simulink library "Valeo_Simulink_Library_EC"  (R2017b)
settings: Solver=ode45  StartTime=0.0  StopTime=10.0  RelTol=1e-3  EnableMultiTasking=on
undefined symbols (not defined in the file): A, B, C, Count_Max, D, InitValue, j, ke, kf, kt, L, Length, MaxIniVal, MaxVal, MinVal, NumBits1, NumBits2, P, p0, Q, R, Simulink_Library, Ts, x0
libraries: Valeo_Simulink_Library_EC x9, simulink x8, fixpt_dtprop x4
(part 2 of 3)

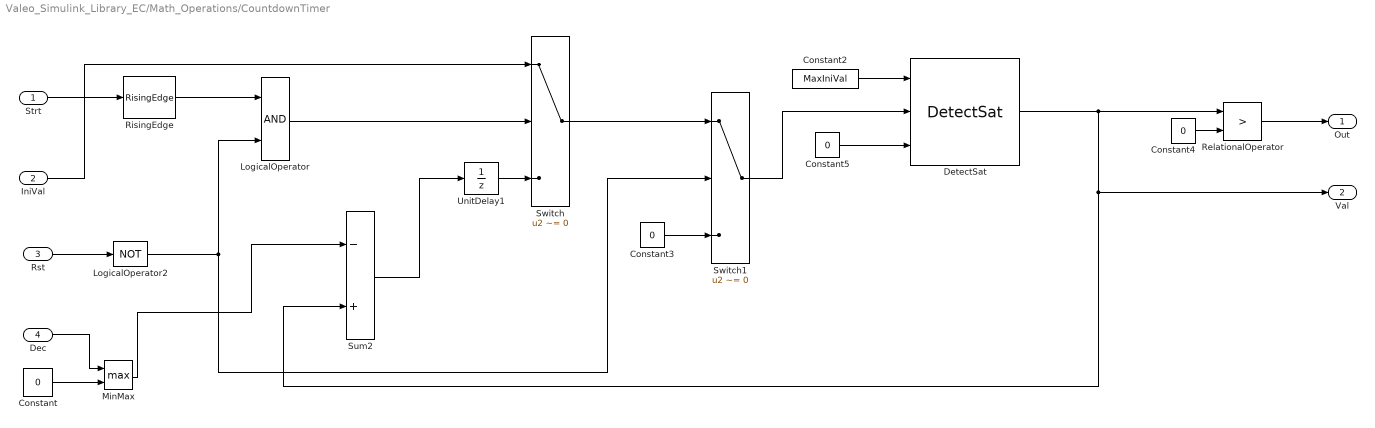
== system Valeo_Simulink_Library_EC/Math_Operations/CountdownTimer ==
  Strt : Inport
  IniVal : Inport  Port=2
  Rst : Inport  Port=3
  Dec : Inport  Port=4
  Constant : Constant  Value=0  OutDataTypeStr=Inherit: Inherit via back propagation
  Constant2 : Constant  Value=MaxIniVal  OutDataTypeStr=Inherit: Inherit via back propagation  SampleTime=-1
  Constant3 : Constant  Value=0  OutDataTypeStr=Inherit: Inherit via back propagation  SampleTime=-1
  Constant4 : Constant  Value=0  OutDataTypeStr=Inherit: Inherit via back propagation  SampleTime=-1
  Constant5 : Constant  Value=0  OutDataTypeStr=Inherit: Inherit via back propagation  SampleTime=-1
  DetectSat : Valeo_Simulink_Library_EC/Signal_Operations/DetectSat  FlagHitMax=off  FlagHitMin=off  FlagOut=on  FlagRevThr=off  EnableRevThreshold=No  LibType=Simulink_Library
  LogicalOperator : Logic  OutDataTypeStr=boolean
  LogicalOperator2 : Logic  Operator=NOT  Inputs=3  OutDataTypeStr=boolean
  MinMax : MinMax  Function=max  Inputs=2  InputSameDT=on
  RelationalOperator : RelationalOperator  Operator=>  OutDataTypeStr=boolean  RndMeth=Nearest  InputSameDT=on
  RisingEdge : Valeo_Simulink_Library_EC/Signal_Operations/RisingEdge  INIT=0
  Sum2 : Sum  Inputs=-+  OutDataTypeStr=Inherit: Inherit via back propagation  RndMeth=Nearest  SaturateOnIntegerOverflow=on  InputSameDT=on
  Switch : Switch  Tag=struct('comment',struct('text','','placement',1),'logdata',struct('maxnumvals',inf,'plotchannels',[],'loggingmode',3,'channels',1),'output',struct('variable','','description','','name','$S_$B','width',1,'address','','max',NaN,'min',NaN,'class','default','type','CONTINUOUS','scaling','','lsb',1,'offset',0,'arb',0,'freeze',1,'unit','','autoscalingmode',1,'lowerheadroom',1,'upperheadroom',1,'headroomunit','bit','keepdatatype',1,'checkmin',0,'checkmax',0,'castoutput',0,'show',0),'threshold',struct('variable','','description','','name','$S_$B_threshold','width',1,'address','','max',NaN,'min',NaN,'class','default','type','CONTINUOUS','scaling','','lsb',1,'offset',0,'arb',0,'freeze',1,'unit','','keepdatatype',1,'value','0','scalar',0,'criteria',3),'scalingvalid',0,'date',733087.49614628474,'inheritscaling',0)  Criteria=u2 ~= 0  OutDataTypeStr=Inherit: Inherit via back propagation  RndMeth=Nearest  SaturateOnIntegerOverflow=on  InputSameDT=on
      settings: AttributesFormatString=threshold=%<threshold>\nCriteria : %<Criteria>
  Switch1 : Switch  Tag=struct('comment',struct('text','','placement',1),'logdata',struct('maxnumvals',inf,'plotchannels',[],'loggingmode',3,'channels',1),'output',struct('variable','','description','','name','$S_$B','width',1,'address','','max',NaN,'min',NaN,'class','default','type','CONTINUOUS','scaling','','lsb',1,'offset',0,'arb',0,'freeze',1,'unit','','autoscalingmode',1,'lowerheadroom',1,'upperheadroom',1,'headroomunit','bit','keepdatatype',1,'checkmin',0,'checkmax',0,'castoutput',0,'show',0),'threshold',struct('variable','','description','','name','$S_$B_threshold','width',1,'address','','max',NaN,'min',NaN,'class','default','type','CONTINUOUS','scaling','','lsb',1,'offset',0,'arb',0,'freeze',1,'unit','','keepdatatype',1,'value','0','scalar',0,'criteria',3),'scalingvalid',0,'date',733087.49614628474,'inheritscaling',0)  Criteria=u2 ~= 0  RndMeth=Nearest  SaturateOnIntegerOverflow=on  InputSameDT=on
      settings: AttributesFormatString=threshold=%<threshold>\nCriteria : %<Criteria>
  UnitDelay1 : UnitDelay  SampleTime=-1
      settings: AttributesFormatString=%<Name>\nTe = %<SampleTime>\nIni=%<X0>
  Out : Outport
  Val : Outport  Port=2
  wires:
  Constant/1 -> MinMax/2
  Constant5/1 -> DetectSat/3
  Constant4/1 -> RelationalOperator/2
  UnitDelay1/1 -> Switch/3
  DetectSat/1 -> Val/1, Sum2/2, RelationalOperator/1
  IniVal/1 -> Switch/1
  LogicalOperator/1 -> Switch/2
  Rst/1 -> LogicalOperator2/1
  RelationalOperator/1 -> Out/1
  Strt/1 -> RisingEdge/1
  RisingEdge/1 -> LogicalOperator/1
  LogicalOperator2/1 -> Switch1/2, LogicalOperator/2
  Constant3/1 -> Switch1/3
  Switch/1 -> Switch1/1
  Dec/1 -> MinMax/1
  Constant2/1 -> DetectSat/1
  Switch1/1 -> DetectSat/2
  MinMax/1 -> Sum2/1
  Sum2/1 -> UnitDelay1/1

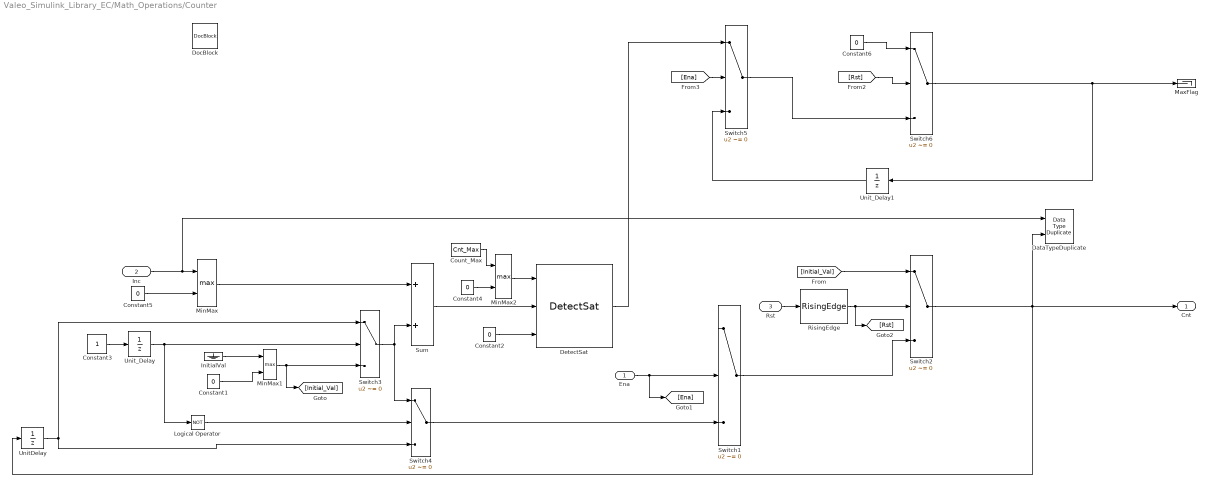
== system Valeo_Simulink_Library_EC/Math_Operations/Counter ==
  Ena : Inport  OutDataTypeStr=boolean
  Inc : Inport  Port=2
  Rst : Inport  Port=3
  Constant{1..2,4..6} (5 alike) : Constant  Value=0  OutDataTypeStr=Inherit: Inherit via back propagation  SampleTime=-1
  Constant3 : Constant  OutDataTypeStr=boolean  SampleTime=-1
  Count_Max : Constant  Value=Cnt_Max
  DataTypeDuplicate : DataTypeDuplicate
  DetectSat : Valeo_Simulink_Library_EC/Signal_Operations/DetectSat  RequirementInfo={} %GIDa_9bb61fc0_0d7a_4d30_bf11_8496912d343b  FlagHitMax=on  FlagHitMin=off  FlagOut=on  FlagRevThr=off  EnableRevThreshold=Yes  LibType=Simulink_Library
  DocBlock : simulink/Model-Wide Utilities/DocBlock  DocumentType=Text
      content=|
      | Block Name: Counter
      |
      | Description:
      | Count up block optional inputs and outputs as per the needed application.
      | "Ena" inport and "Cnt" outport are mandatory.
      | "Inc", "Rst", "InitialVal" and "Count_Max" are optional inports.
      | "MaxFlag" is an optional outport.
      | If "Inc" is not selected from the mask, default increment step is 1.
      | If "Rst" is not selected from the mask, the port is grounded.
      | If "InitialVal" is not selected from the mask, default initial value is 0.
      | If "Count_Max" is not selected from the mask, the value has to be entered
      | from the mask itself as a parameter.
      | If "MaxFlag" is not selected from the mask, the port is terminated.
      |
      | Requirements Document:VIAS_T02_15_019_Valeo_Simulink_Library_SRS
      |                       Section:5.1.4
      |
      | Last Edit made by: sahmed1 on 17/3/2019
      |
      | Block Version: 1.1
  InitialVal : Ground
  Logical Operator : Logic  Operator=NOT  AllPortsSameDT=off  OutDataTypeStr=boolean
  MaxFlag : Terminator
  MinMax : MinMax  RequirementInfo={} %GIDa_05f1e69c_f4c8_4dbb_8851_ae441f19c864  Function=max  Inputs=2  OutDataTypeStr=Inherit: Inherit via back propagation  ZeroCross=off  SaturateOnIntegerOverflow=on  InputSameDT=on
  MinMax1 : MinMax  Function=max  Inputs=2  OutDataTypeStr=Inherit: Inherit via back propagation  ZeroCross=off  SaturateOnIntegerOverflow=on  InputSameDT=on
  MinMax2 : MinMax  Function=max  Inputs=2  OutDataTypeStr=Inherit: Inherit via back propagation  ZeroCross=off  SaturateOnIntegerOverflow=on  InputSameDT=on
  RisingEdge : Valeo_Simulink_Library_EC/Signal_Operations/RisingEdge  RequirementInfo={} %GIDa_9731123e_4d8d_47b4_b498_60fb13b5864c  INIT=0
  Sum : Sum  RequirementInfo={} %GIDa_8f895930_75b4_4d04_b64c_37162e5979c7  OutDataTypeStr=Inherit: Inherit via back propagation  SaturateOnIntegerOverflow=on  InputSameDT=on
  Switch1 : Switch  Tag=struct('comment',struct('text','','placement',1),'logdata',struct('maxnumvals',inf,'plotchannels',[],'loggingmode',3,'channels',1),'output',struct('variable','','description','','name','$S_$B','width',1,'address','','max',NaN,'min',NaN,'class','default','type','CONTINUOUS','scaling','','lsb',1,'offset',0,'arb',0,'freeze',1,'unit','','autoscalingmode',1,'lowerheadroom',1,'upperheadroom',1,'headroomunit','bit','keepdatatype',1,'checkmin',0,'checkmax',0,'castoutput',0,'show',0),'threshold',struct('variable','','description','','name','$S_$B_threshold','width',1,'address','','max',NaN,'min',NaN,'class','default','type','CONTINUOUS','scaling','','lsb',1,'offset',0,'arb',0,'freeze',1,'unit','','keepdatatype',1,'value','0','scalar',0,'criteria',3),'scalingvalid',0,'date',733087.49614628474,'inheritscaling',0)  RequirementInfo={} %GIDa_3188b40d_7524_43cd_a4e7_8fa433184620  Criteria=u2 ~= 0  ZeroCross=off  InputSameDT=on
      settings: AttributesFormatString=threshold=%<threshold>\nCriteria : %<Criteria>
  Switch2 : Switch  Tag=struct('comment',struct('text','','placement',1),'logdata',struct('maxnumvals',inf,'plotchannels',[],'loggingmode',3,'channels',1),'output',struct('variable','','description','','name','$S_$B','width',1,'address','','max',NaN,'min',NaN,'class','default','type','CONTINUOUS','scaling','','lsb',1,'offset',0,'arb',0,'freeze',1,'unit','','autoscalingmode',1,'lowerheadroom',1,'upperheadroom',1,'headroomunit','bit','keepdatatype',1,'checkmin',0,'checkmax',0,'castoutput',0,'show',0),'threshold',struct('variable','','description','','name','$S_$B_threshold','width',1,'address','','max',NaN,'min',NaN,'class','default','type','CONTINUOUS','scaling','','lsb',1,'offset',0,'arb',0,'freeze',1,'unit','','keepdatatype',1,'value','0','scalar',0,'criteria',3),'scalingvalid',0,'date',733087.49614628474,'inheritscaling',0)  RequirementInfo={} %GIDa_e3ab621a_27e3_4b82_bf67_d379718e39ab  Criteria=u2 ~= 0  OutDataTypeStr=Inherit: Inherit via back propagation  ZeroCross=off  InputSameDT=on
      settings: AttributesFormatString=threshold=%<threshold>\nCriteria : %<Criteria>
  Switch3 : Switch  RequirementInfo={} %GIDa_6adc28a8_417c_42d0_96f8_0bd9c0ac3dfc  Criteria=u2 ~= 0  RndMeth=Nearest  InputSameDT=on
      settings: AttributesFormatString=Cond=%<Criteria>\nThreshold=%<Threshold>
  Switch4 : Switch  RequirementInfo={} %GIDa_4bec96d5_6195_44e1_b82b_bfaee5774d71  Criteria=u2 ~= 0  RndMeth=Nearest  InputSameDT=on
      settings: AttributesFormatString=Cond=%<Criteria>\nThreshold=%<Threshold>
  Switch5 : Switch  Tag=struct('comment',struct('text','','placement',1),'logdata',struct('maxnumvals',inf,'plotchannels',[],'loggingmode',3,'channels',1),'output',struct('variable','','description','','name','$S_$B','width',1,'address','','max',NaN,'min',NaN,'class','default','type','CONTINUOUS','scaling','','lsb',1,'offset',0,'arb',0,'freeze',1,'unit','','autoscalingmode',1,'lowerheadroom',1,'upperheadroom',1,'headroomunit','bit','keepdatatype',1,'checkmin',0,'checkmax',0,'castoutput',0,'show',0),'threshold',struct('variable','','description','','name','$S_$B_threshold','width',1,'address','','max',NaN,'min',NaN,'class','default','type','CONTINUOUS','scaling','','lsb',1,'offset',0,'arb',0,'freeze',1,'unit','','keepdatatype',1,'value','0','scalar',0,'criteria',3),'scalingvalid',0,'date',733087.49614628474,'inheritscaling',0)  RequirementInfo={} %GIDa_5a250cc1_c600_4491_b832_9bb443b73e74  Criteria=u2 ~= 0  ZeroCross=off  InputSameDT=on
      settings: AttributesFormatString=threshold=%<threshold>\nCriteria : %<Criteria>
  Switch6 : Switch  Tag=struct('comment',struct('text','','placement',1),'logdata',struct('maxnumvals',inf,'plotchannels',[],'loggingmode',3,'channels',1),'output',struct('variable','','description','','name','$S_$B','width',1,'address','','max',NaN,'min',NaN,'class','default','type','CONTINUOUS','scaling','','lsb',1,'offset',0,'arb',0,'freeze',1,'unit','','autoscalingmode',1,'lowerheadroom',1,'upperheadroom',1,'headroomunit','bit','keepdatatype',1,'checkmin',0,'checkmax',0,'castoutput',0,'show',0),'threshold',struct('variable','','description','','name','$S_$B_threshold','width',1,'address','','max',NaN,'min',NaN,'class','default','type','CONTINUOUS','scaling','','lsb',1,'offset',0,'arb',0,'freeze',1,'unit','','keepdatatype',1,'value','0','scalar',0,'criteria',3),'scalingvalid',0,'date',733087.49614628474,'inheritscaling',0)  RequirementInfo={} %GIDa_72ede8d6_7b52_4ad1_ab42_e02456330975  Criteria=u2 ~= 0  OutDataTypeStr=Inherit: Inherit via back propagation  ZeroCross=off  InputSameDT=on
      settings: AttributesFormatString=threshold=%<threshold>\nCriteria : %<Criteria>
  UnitDelay : UnitDelay  SampleTime=-1
      settings: AttributesFormatString=%<Name>\nTe = %<SampleTime>\nIni=%<X0>
  Unit_Delay : UnitDelay  SampleTime=-1
  Unit_Delay1 : UnitDelay  SampleTime=-1
  Cnt : Outport  RequirementInfo={} %GIDa_ced6db0b_0aef_4b74_b197_441398289d0b
  wires:
  Switch5/1 -> Switch6/3
  Constant6/1 -> Switch6/1
  Unit_Delay1/1 -> Switch5/3
  [Ena] -> Switch5/2
  DetectSat/1 -> Switch5/1
  [Rst] -> Switch6/2
  Rst/1 -> RisingEdge/1
  ? -> Switch1/1
  Switch6/1 -> Unit_Delay1/1, MaxFlag/1
  Sum/1 -> DetectSat/2
  Count_Max/1 -> MinMax2/1
  MinMax2/1 -> DetectSat/1
  InitialVal/1 -> MinMax1/1
  MinMax1/1 -> Switch3/3, [Initial_Val]
  Constant1/1 -> MinMax1/2
  Constant4/1 -> MinMax2/2
  Switch1/1 -> Switch2/3
  MinMax/1 -> Sum/1
  Unit_Delay/1 -> Logical Operator/1, Switch3/2
  Constant3/1 -> Unit_Delay/1
  Switch3/1 -> Switch4/1, Sum/2
  Inc/1 -> MinMax/1, DataTypeDuplicate/1
  RisingEdge/1 -> Switch2/2, [Rst]
  Constant5/1 -> MinMax/2
  Constant2/1 -> DetectSat/3
  Ena/1 -> Switch1/2, [Ena]
  Switch4/1 -> Switch1/3
  Logical Operator/1 -> Switch4/2
  Switch2/1 -> DataTypeDuplicate/2, Cnt/1, UnitDelay/1
  UnitDelay/1 -> Switch4/3, Switch3/1
  [Initial_Val] -> Switch2/1

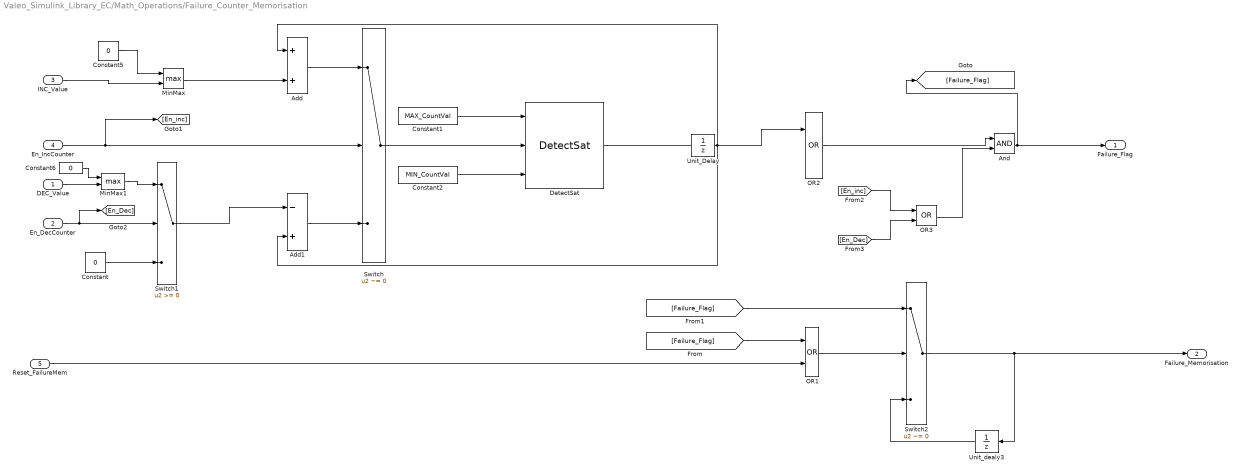
== system Valeo_Simulink_Library_EC/Math_Operations/Failure_Counter_Memorisation ==
  DEC_Value : Inport
  En_DecCounter : Inport  Port=2  OutDataTypeStr=boolean
  INC_Value : Inport  Port=3
  En_IncCounter : Inport  Port=4  OutDataTypeStr=boolean
  Reset_FailureMem : Inport  Port=5  OutDataTypeStr=boolean
  Add : Sum
  Add1 : Sum  Inputs=-+
  And : Logic  AllPortsSameDT=off  OutDataTypeStr=boolean
  Constant : Constant  Value=0  OutDataTypeStr=Inherit: Inherit via back propagation
  Constant1 : Constant  Value=MAX_CountVal
  Constant2 : Constant  Value=MIN_CountVal
  Constant5 : Constant  Value=0  OutDataTypeStr=Inherit: Inherit via back propagation
  Constant6 : Constant  Value=0  OutDataTypeStr=Inherit: Inherit via back propagation
  DetectSat : Valeo_Simulink_Library_EC/Signal_Operations/DetectSat  Description=DetectSat  RequirementInfo={} %GIDa_f7c90ce4_a1b3_4851_83d7_a18600e936e6  FlagHitMax=on  FlagHitMin=on  FlagOut=on  FlagRevThr=off  EnableRevThreshold=No  LibType=Simulink_Library
  MinMax : MinMax  Function=max  Inputs=2
  MinMax1 : MinMax  Function=max  Inputs=2
  OR1 : Logic  RequirementInfo={} %GIDa_04208e23_291f_48af_9c39_d5bad472f985  Operator=OR  AllPortsSameDT=off  OutDataTypeStr=boolean
  OR2 : Logic  RequirementInfo={} %GIDa_9651d414_1c4d_4a50_8930_c47158f8b0f5  Operator=OR  AllPortsSameDT=off  OutDataTypeStr=boolean
  OR3 : Logic  Operator=OR  AllPortsSameDT=off  OutDataTypeStr=boolean
  Switch : Switch  RequirementInfo={} %GIDa_288fa2ec_3de0_4803_93ac_92640899949d  Criteria=u2 ~= 0
  Switch1 : Switch
  Switch2 : Switch  RequirementInfo={} %GIDa_0183bc51_af57_411f_b819_c082a7e6d6c2  Criteria=u2 ~= 0
  Unit_Delay : UnitDelay  SampleTime=-1
  Unit_dealy3 : UnitDelay  SampleTime=-1
  Failure_Flag : Outport  Tag=AM,Out,1,0,Name,NC;CMP,Port,OutputWhenDisabled,InitialOutput;  OutDataTypeStr=boolean
      settings: AttributesFormatString=%<OutputWhenDisabled>\n%<InitialOutput>\n
  Failure_Memorisation : Outport  Port=2  OutDataTypeStr=boolean
  wires:
  [Failure_Flag] -> OR1/1
  [Failure_Flag] -> Switch2/1
  Unit_dealy3/1 -> Switch2/3
  OR1/1 -> Switch2/2
  Switch2/1 -> Unit_dealy3/1, Failure_Memorisation/1
  Reset_FailureMem/1 -> OR1/2
  En_IncCounter/1 -> Switch/2, [En_inc]
  MinMax/1 -> Add/2
  INC_Value/1 -> MinMax/2
  Add/1 -> Switch/1
  Unit_Delay/1 -> Add/1, Add1/2
  Switch1/1 -> Add1/1
  Constant/1 -> Switch1/3
  En_DecCounter/1 -> [En_Dec], Switch1/2
  MinMax1/1 -> Switch1/1
  Constant6/1 -> MinMax1/1
  DEC_Value/1 -> MinMax1/2
  Add1/1 -> Switch/3
  And/1 -> [Failure_Flag], Failure_Flag/1
  OR2/1 -> And/1
  OR3/1 -> And/2
  [En_Dec] -> OR3/2
  [En_inc] -> OR3/1
  Constant5/1 -> MinMax/1
  Constant2/1 -> DetectSat/3
  Constant1/1 -> DetectSat/1
  Switch/1 -> DetectSat/2
  DetectSat/1 -> OR2/1
  ? -> OR2/2
  ? -> Unit_Delay/1

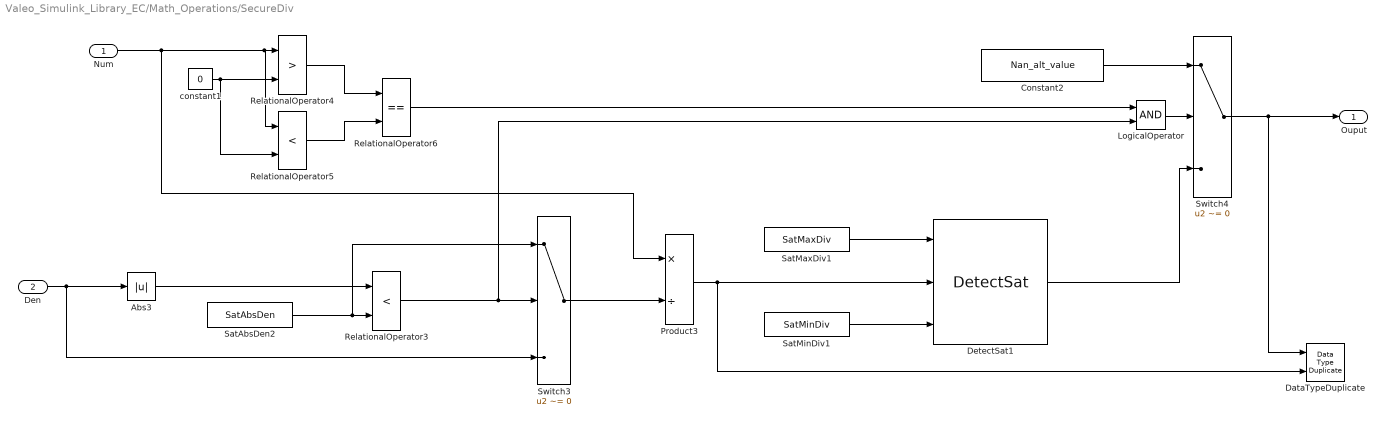
== system Valeo_Simulink_Library_EC/Math_Operations/SecureDiv ==
  Num : Inport
  Den : Inport  Port=2
  Abs3 : Abs  SaturateOnIntegerOverflow=on
  Constant2 : Constant  Value=Nan_alt_value  OutDataTypeStr=Inherit: Inherit via back propagation  SampleTime=-1  LockScale=on
  DataTypeDuplicate : DataTypeDuplicate
  DetectSat1 : Valeo_Simulink_Library_EC/Signal_Operations/DetectSat  FlagHitMax=off  FlagHitMin=off  FlagOut=on  FlagRevThr=off  EnableRevThreshold=No  LibType=Simulink_Library
  LogicalOperator : Logic  AllPortsSameDT=off  OutDataTypeStr=boolean
  Product3 : Product  Tag=struct('comment',struct('text','','placement',1),'logdata',struct('maxnumvals',inf,'plotchannels',[],'loggingmode',3,'channels',1),'output',struct('variable','','description','','name','$S_$B','width',1,'address','','max',NaN,'min',NaN,'class','default','type','CONTINUOUS','scaling','','lsb',1,'offset',0,'arb',0,'freeze',1,'unit','','autoscalingmode',1,'lowerheadroom',1,'upperheadroom',1,'headroomunit','bit','keepdatatype',1,'checkmin',0,'checkmax',0,'castoutput',0,'show',0),'inputs','**','exceptionhandling',1,'scalingvalid',0,'date',730486)  Inputs=*/  OutDataTypeStr=Inherit: Inherit via back propagation  RndMeth=Nearest  SaturateOnIntegerOverflow=on
  RelationalOperator3 : RelationalOperator  Operator=<  OutDataTypeStr=boolean  RndMeth=Nearest  InputSameDT=on
  RelationalOperator4 : RelationalOperator  Operator=>  OutDataTypeStr=boolean  RndMeth=Nearest  InputSameDT=on
  RelationalOperator5 : RelationalOperator  Operator=<  OutDataTypeStr=boolean  RndMeth=Nearest  InputSameDT=on
  RelationalOperator6 : RelationalOperator  Operator===  OutDataTypeStr=boolean  RndMeth=Nearest  InputSameDT=on
  SatAbsDen2 : Constant  Tag=struct('comment',struct('text','','placement',1),'output',struct('variable','','description','','name','$S_$B','width',1,'address','','max',NaN,'min',NaN,'class','default','type','CONTINUOUS','scaling','','lsb',1,'offset',0,'arb',0,'freeze',1,'unit','','keepdatatype',1,'value','1','tolerance',1,'castoutput',0,'show',0),'dt','inf','scalingvalid',0,'date',730486)  Value=SatAbsDen  OutDataTypeStr=Inherit: Inherit via back propagation  SampleTime=-1
  SatMaxDiv1 : Constant  Tag=struct('comment',struct('text','','placement',1),'output',struct('variable','','description','','name','$S_$B','width',1,'address','','max',NaN,'min',NaN,'class','default','type','CONTINUOUS','scaling','','lsb',1,'offset',0,'arb',0,'freeze',1,'unit','','keepdatatype',1,'value','1','tolerance',1,'castoutput',0,'show',0),'dt','inf','scalingvalid',0,'date',730486)  Value=SatMaxDiv  OutDataTypeStr=Inherit: Inherit via back propagation  SampleTime=-1
  SatMinDiv1 : Constant  Tag=struct('comment',struct('text','','placement',1),'output',struct('variable','','description','','name','$S_$B','width',1,'address','','max',NaN,'min',NaN,'class','default','type','CONTINUOUS','scaling','','lsb',1,'offset',0,'arb',0,'freeze',1,'unit','','keepdatatype',1,'value','1','tolerance',1,'castoutput',0,'show',0),'dt','inf','scalingvalid',0,'date',730486)  Value=SatMinDiv  OutDataTypeStr=Inherit: Inherit via back propagation  SampleTime=-1
  Switch3 : Switch  Tag=struct('comment',struct('text','','placement',1),'logdata',struct('maxnumvals',inf,'plotchannels',[],'loggingmode',3,'channels',1),'output',struct('variable','','description','','name','$S_$B','width',1,'address','','max',NaN,'min',NaN,'class','default','type','CONTINUOUS','scaling','','lsb',1,'offset',0,'arb',0,'freeze',1,'unit','','autoscalingmode',1,'lowerheadroom',1,'upperheadroom',1,'headroomunit','bit','keepdatatype',1,'checkmin',0,'checkmax',0,'castoutput',0,'show',0),'threshold',struct('variable','','description','','name','$S_$B_threshold','width',1,'address','','max',NaN,'min',NaN,'class','default','type','CONTINUOUS','scaling','','lsb',1,'offset',0,'arb',0,'freeze',1,'unit','','keepdatatype',1,'value','0','scalar',0,'criteria',3),'scalingvalid',0,'date',733087.49614628474,'inheritscaling',0)  Criteria=u2 ~= 0  SaturateOnIntegerOverflow=on  InputSameDT=on
      settings: AttributesFormatString=threshold=%<threshold>\nCriteria : %<Criteria>
  Switch4 : Switch  Criteria=u2 ~= 0  OutDataTypeStr=Inherit: Inherit via back propagation  RndMeth=Nearest  InputSameDT=on
  constant1 : Constant  Tag=struct('comment',struct('text','','placement',1),'output',struct('variable','','description','','name','$S_$B','width',1,'address','','max',NaN,'min',NaN,'class','default','type','CONTINUOUS','scaling','','lsb',1,'offset',0,'arb',0,'freeze',1,'unit','','keepdatatype',1,'value','1','tolerance',1,'castoutput',0,'show',0),'dt','inf','scalingvalid',0,'date',730486)  Value=0  OutDataTypeStr=Inherit: Inherit via back propagation  SampleTime=-1
  Ouput : Outport
  wires:
  DetectSat1/1 -> Switch4/3
  LogicalOperator/1 -> Switch4/2
  RelationalOperator6/1 -> LogicalOperator/1
  Switch4/1 -> Ouput/1, DataTypeDuplicate/1
  Constant2/1 -> Switch4/1
  RelationalOperator5/1 -> RelationalOperator6/2
  RelationalOperator4/1 -> RelationalOperator6/1
  constant1/1 -> RelationalOperator5/2, RelationalOperator4/2
  Num/1 -> RelationalOperator5/1, RelationalOperator4/1, Product3/1
  SatMaxDiv1/1 -> DetectSat1/1
  SatMinDiv1/1 -> DetectSat1/3
  Product3/1 -> DetectSat1/2, DataTypeDuplicate/2
  SatAbsDen2/1 -> RelationalOperator3/2, Switch3/1
  Switch3/1 -> Product3/2
  RelationalOperator3/1 -> Switch3/2, LogicalOperator/2
  Abs3/1 -> RelationalOperator3/1
  Den/1 -> Switch3/3, Abs3/1

== system Valeo_Simulink_Library_EC/Plant Models/Actuators ==
  BLDC : Subsystem  mask(VSL_BLDC){R=R, L=L, j=j, P=P, ke=ke, kt=kt, kf=kf, x0=x0}
      mask help: BLDC motor model simulates the machine speed, torque and stator currents stimulated by the phase to phase voltage and load torque, assuming trapezoidal back emf.
      mask Display:
      | plot(0,0,100,100)
      | patch(100*[0.88 0.93 0.94 0.99 0.98 0.94 0.9 0.88], 100*[0.11 0.01 0.01 0.11 0.11 0.026 0.11 0.11], [0 1 0])

== system Valeo_Simulink_Library_EC/Plant Models/Sensors ==

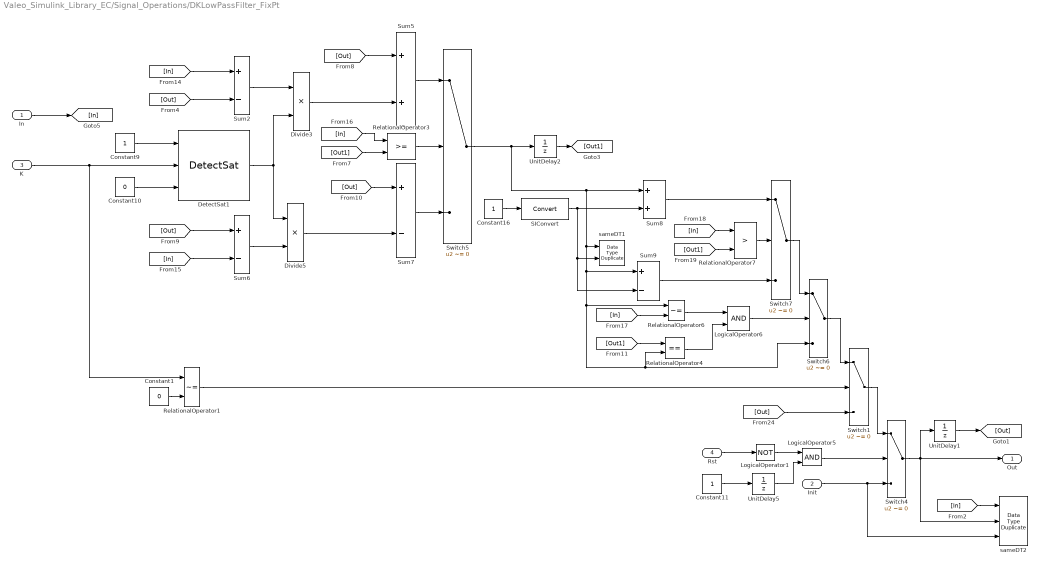
== system Valeo_Simulink_Library_EC/Signal_Operations/DKLowPassFilter_FixPt ==
  In : Inport  RequirementInfo={} %GIDa_0413d053_4ec8_42c5_b371_a8047b2200f3
  Init : Inport  RequirementInfo={} %GIDa_5872fcc3_05fb_45f2_9bed_09235c6b0cac  Port=2
  K : Inport  RequirementInfo={} %GIDa_98114ef1_cbe3_4be6_8894_0cd40cae6f0b  Port=3
  Rst : Inport  RequirementInfo={} %GIDa_1420b06f_654a_4f9a_a3af_ddfdee9c425a  Port=4
  Constant1 : Constant  Value=0  OutDataTypeStr=Inherit: Inherit via back propagation  SampleTime=-1
  Constant10 : Constant  RequirementInfo={} %GIDa_3973ca9d_f818_47df_80ed_9838d1273ef8  Value=0  OutDataTypeStr=Inherit: Inherit via back propagation  SampleTime=-1
  Constant11 : Constant  RequirementInfo={} %GIDa_d28a1eeb_ec69_477b_bb73_5596cd9e0263  OutDataTypeStr=boolean  SampleTime=-1
  Constant16 : Constant  RequirementInfo={} %GIDa_6d10a8d6_24a5_4fbd_9218_f05ddc57d3c3  OutDataTypeStr=uint8  SampleTime=-1
  Constant9 : Constant  RequirementInfo={} %GIDa_f21fb39a_79b6_494f_8e0c_3ee289bd9826  OutDataTypeStr=Inherit: Inherit via back propagation  SampleTime=-1
  DetectSat1 : Valeo_Simulink_Library_EC/Signal_Operations/DetectSat  RequirementInfo={} %GIDa_5313b4e0_40e1_4e21_9a31_65be49b89e34  FlagHitMax=off  FlagHitMin=off  FlagOut=on  FlagRevThr=off  EnableRevThreshold=No  LibType=Simulink_Library
  Divide3 : Product  Tag=struct('comment',struct('text','','placement',1),'logdata',struct('maxnumvals',inf,'plotchannels',[],'loggingmode',3,'channels',1),'output',struct('variable','','description','','name','$S_$B','width',1,'address','','max',NaN,'min',NaN,'class','default','type','CONTINUOUS','scaling','','lsb',1,'offset',0,'arb',0,'freeze',1,'unit','','autoscalingmode',1,'lowerheadroom',1,'upperheadroom',1,'headroomunit','bit','keepdatatype',1,'checkmin',0,'checkmax',0,'castoutput',0,'show',0),'inputs','**','exceptionhandling',1,'scalingvalid',0,'date',730486)  RequirementInfo={} %GIDa_0415ca49_d04f_4698_b9e2_db1e83986d60  Inputs=**  RndMeth=Simplest  SaturateOnIntegerOverflow=on
  Divide5 : Product  Tag=struct('comment',struct('text','','placement',1),'logdata',struct('maxnumvals',inf,'plotchannels',[],'loggingmode',3,'channels',1),'output',struct('variable','','description','','name','$S_$B','width',1,'address','','max',NaN,'min',NaN,'class','default','type','CONTINUOUS','scaling','','lsb',1,'offset',0,'arb',0,'freeze',1,'unit','','autoscalingmode',1,'lowerheadroom',1,'upperheadroom',1,'headroomunit','bit','keepdatatype',1,'checkmin',0,'checkmax',0,'castoutput',0,'show',0),'inputs','**','exceptionhandling',1,'scalingvalid',0,'date',730486)  RequirementInfo={} %GIDa_3f77597f_4279_4430_aaf5_1f9e615d91c4  Inputs=**  RndMeth=Simplest  SaturateOnIntegerOverflow=on
  LogicalOperator1 : Logic  RequirementInfo={} %GIDa_2177e6af_1734_40b8_84ff_f9a943bf7bd3  Operator=NOT  Inputs=1  OutDataTypeStr=boolean
  LogicalOperator5 : Logic  RequirementInfo={} %GIDa_152c7f3e_4ce8_481e_b7cc_9fb4cf693d00  OutDataTypeStr=boolean
  LogicalOperator6 : Logic  RequirementInfo={} %GIDa_d1fafc81_c9e4_4943_bea4_15d197491b3a  OutDataTypeStr=boolean
  RelationalOperator1 : RelationalOperator  Operator=~=  OutDataTypeStr=boolean  RndMeth=Nearest  InputSameDT=on
  RelationalOperator3 : RelationalOperator  RequirementInfo={} %GIDa_977d0204_36a9_4c5d_b531_b2483a36d0fb  OutDataTypeStr=boolean  RndMeth=Nearest
  RelationalOperator4 : RelationalOperator  RequirementInfo={} %GIDa_5315e60a_98f0_4e80_a073_c68638eac179  Operator===  OutDataTypeStr=boolean  RndMeth=Nearest  InputSameDT=on
  RelationalOperator6 : RelationalOperator  RequirementInfo={} %GIDa_e57606ca_fa40_4915_aca9_16f2019bccb7  Operator=~=  OutDataTypeStr=boolean  RndMeth=Nearest  InputSameDT=on
  RelationalOperator7 : RelationalOperator  RequirementInfo={} %GIDa_1a441538_5fa6_4ce2_b169_6eab377cb876  Operator=>  OutDataTypeStr=boolean  RndMeth=Nearest
  SIConvert : DataTypeConversion  RequirementInfo={} %GIDa_4d226239_20ca_4daf_9af1_a668e13d4201  ConvertRealWorld=Stored Integer (SI)  RndMeth=Simplest
  Sum2 : Sum  RequirementInfo={} %GIDa_16df61f3_54b0_441a_a749_ffaba2d118b6  Inputs=+-  RndMeth=Nearest  SaturateOnIntegerOverflow=on  InputSameDT=on  OutDataTypeStr=Inherit: Same as first input
  Sum5 : Sum  RequirementInfo={} %GIDa_3659f147_b6d6_44ef_bd32_19e97590d9e6  OutDataTypeStr=Inherit: Inherit via back propagation  RndMeth=Nearest
  Sum6 : Sum  RequirementInfo={} %GIDa_0be8a480_2cfa_4e15_923a_a98cce8241cf  Inputs=+-  RndMeth=Nearest  SaturateOnIntegerOverflow=on  InputSameDT=on  OutDataTypeStr=Inherit: Same as first input
  Sum7 : Sum  RequirementInfo={} %GIDa_a6bb31c3_1de1_4b77_a2ee_1a031954c06f  Inputs=+-  RndMeth=Nearest
  Sum8 : Sum  RequirementInfo={} %GIDa_a63f4772_0e99_449a_a004_2693c637ec25  RndMeth=Nearest  SaturateOnIntegerOverflow=on  InputSameDT=on  OutDataTypeStr=Inherit: Same as first input
  Sum9 : Sum  RequirementInfo={} %GIDa_5e0e12b5_0a8c_42a3_9910_9005c0a65fa1  Inputs=+-  RndMeth=Nearest  SaturateOnIntegerOverflow=on  InputSameDT=on  OutDataTypeStr=Inherit: Same as first input
  Switch1 : Switch  Tag=struct('comment',struct('text','','placement',1),'logdata',struct('maxnumvals',inf,'plotchannels',[],'loggingmode',3,'channels',1),'output',struct('variable','','description','','name','$S_$B','width',1,'address','','max',NaN,'min',NaN,'class','default','type','CONTINUOUS','scaling','','lsb',1,'offset',0,'arb',0,'freeze',1,'unit','','autoscalingmode',1,'lowerheadroom',1,'upperheadroom',1,'headroomunit','bit','keepdatatype',1,'checkmin',0,'checkmax',0,'castoutput',0,'show',0),'threshold',struct('variable','','description','','name','$S_$B_threshold','width',1,'address','','max',NaN,'min',NaN,'class','default','type','CONTINUOUS','scaling','','lsb',1,'offset',0,'arb',0,'freeze',1,'unit','','keepdatatype',1,'value','0','scalar',0,'criteria',3),'scalingvalid',0,'date',733087.49614628474,'inheritscaling',0)  Criteria=u2 ~= 0  OutDataTypeStr=Inherit: Inherit via back propagation  SaturateOnIntegerOverflow=on  InputSameDT=on
      settings: AttributesFormatString=threshold=%<threshold>\nCriteria : %<Criteria>
  Switch4 : Switch  Tag=struct('comment',struct('text','','placement',1),'logdata',struct('maxnumvals',inf,'plotchannels',[],'loggingmode',3,'channels',1),'output',struct('variable','','description','','name','$S_$B','width',1,'address','','max',NaN,'min',NaN,'class','default','type','CONTINUOUS','scaling','','lsb',1,'offset',0,'arb',0,'freeze',1,'unit','','autoscalingmode',1,'lowerheadroom',1,'upperheadroom',1,'headroomunit','bit','keepdatatype',1,'checkmin',0,'checkmax',0,'castoutput',0,'show',0),'threshold',struct('variable','','description','','name','$S_$B_threshold','width',1,'address','','max',NaN,'min',NaN,'class','default','type','CONTINUOUS','scaling','','lsb',1,'offset',0,'arb',0,'freeze',1,'unit','','keepdatatype',1,'value','0','scalar',0,'criteria',3),'scalingvalid',0,'date',733087.49614628474,'inheritscaling',0)  RequirementInfo={} %GIDa_e47b38d0_f58c_46be_8df4_f8c6a1bd3ffa  Criteria=u2 ~= 0  OutDataTypeStr=Inherit: Inherit via back propagation  SaturateOnIntegerOverflow=on  InputSameDT=on
      settings: AttributesFormatString=threshold=%<threshold>\nCriteria : %<Criteria>
  Switch5 : Switch  Tag=struct('comment',struct('text','','placement',1),'logdata',struct('maxnumvals',inf,'plotchannels',[],'loggingmode',3,'channels',1),'output',struct('variable','','description','','name','$S_$B','width',1,'address','','max',NaN,'min',NaN,'class','default','type','CONTINUOUS','scaling','','lsb',1,'offset',0,'arb',0,'freeze',1,'unit','','autoscalingmode',1,'lowerheadroom',1,'upperheadroom',1,'headroomunit','bit','keepdatatype',1,'checkmin',0,'checkmax',0,'castoutput',0,'show',0),'threshold',struct('variable','','description','','name','$S_$B_threshold','width',1,'address','','max',NaN,'min',NaN,'class','default','type','CONTINUOUS','scaling','','lsb',1,'offset',0,'arb',0,'freeze',1,'unit','','keepdatatype',1,'value','0','scalar',0,'criteria',3),'scalingvalid',0,'date',733087.49614628474,'inheritscaling',0)  RequirementInfo={} %GIDa_305754b4_fced_4041_a2cf_36c9fa36be9d  Criteria=u2 ~= 0  OutDataTypeStr=Inherit: Inherit via back propagation  SaturateOnIntegerOverflow=on  InputSameDT=on
      settings: AttributesFormatString=threshold=%<threshold>\nCriteria : %<Criteria>
  Switch6 : Switch  Tag=struct('comment',struct('text','','placement',1),'logdata',struct('maxnumvals',inf,'plotchannels',[],'loggingmode',3,'channels',1),'output',struct('variable','','description','','name','$S_$B','width',1,'address','','max',NaN,'min',NaN,'class','default','type','CONTINUOUS','scaling','','lsb',1,'offset',0,'arb',0,'freeze',1,'unit','','autoscalingmode',1,'lowerheadroom',1,'upperheadroom',1,'headroomunit','bit','keepdatatype',1,'checkmin',0,'checkmax',0,'castoutput',0,'show',0),'threshold',struct('variable','','description','','name','$S_$B_threshold','width',1,'address','','max',NaN,'min',NaN,'class','default','type','CONTINUOUS','scaling','','lsb',1,'offset',0,'arb',0,'freeze',1,'unit','','keepdatatype',1,'value','0','scalar',0,'criteria',3),'scalingvalid',0,'date',733087.49614628474,'inheritscaling',0)  RequirementInfo={} %GIDa_94e7d435_4b45_4652_8412_fe302bdfd76e  Criteria=u2 ~= 0  OutDataTypeStr=Inherit: Inherit via back propagation  SaturateOnIntegerOverflow=on  InputSameDT=on
      settings: AttributesFormatString=threshold=%<threshold>\nCriteria : %<Criteria>
  Switch7 : Switch  Tag=struct('comment',struct('text','','placement',1),'logdata',struct('maxnumvals',inf,'plotchannels',[],'loggingmode',3,'channels',1),'output',struct('variable','','description','','name','$S_$B','width',1,'address','','max',NaN,'min',NaN,'class','default','type','CONTINUOUS','scaling','','lsb',1,'offset',0,'arb',0,'freeze',1,'unit','','autoscalingmode',1,'lowerheadroom',1,'upperheadroom',1,'headroomunit','bit','keepdatatype',1,'checkmin',0,'checkmax',0,'castoutput',0,'show',0),'threshold',struct('variable','','description','','name','$S_$B_threshold','width',1,'address','','max',NaN,'min',NaN,'class','default','type','CONTINUOUS','scaling','','lsb',1,'offset',0,'arb',0,'freeze',1,'unit','','keepdatatype',1,'value','0','scalar',0,'criteria',3),'scalingvalid',0,'date',733087.49614628474,'inheritscaling',0)  RequirementInfo={} %GIDa_e4174117_20c5_42b6_8eb3_7186d44de704  Criteria=u2 ~= 0  OutDataTypeStr=Inherit: Inherit via back propagation  SaturateOnIntegerOverflow=on  InputSameDT=on
      settings: AttributesFormatString=threshold=%<threshold>\nCriteria : %<Criteria>
  UnitDelay1 : UnitDelay  RequirementInfo={} %GIDa_6cdea363_ef54_4016_8e77_15ded96ef26e  SampleTime=-1
      settings: AttributesFormatString=%<Name>\nTe = %<SampleTime>\nIni=%<X0>
  UnitDelay2 : UnitDelay  RequirementInfo={} %GIDa_b3299467_8f74_4ca2_89ee_edf192f96fae  SampleTime=-1
      settings: AttributesFormatString=%<Name>\nTe = %<SampleTime>\nIni=%<X0>
  UnitDelay5 : UnitDelay  RequirementInfo={} %GIDa_dc1eba62_d931_470a_bb56_5b1eb490c4c6  SampleTime=-1
      settings: AttributesFormatString=Te = %<SampleTime>\nIni=%<X0>
  sameDT1 : DataTypeDuplicate  RequirementInfo={} %GIDa_e890005e_9383_44fa_a2c6_ed3b4fcfea6b  DisableCoverage=on
  sameDT2 : DataTypeDuplicate  RequirementInfo={} %GIDa_6e215ae5_5a7c_4c45_97f5_398da5175dcf  DisableCoverage=on  NumInputPorts=3
  Out : Outport  RequirementInfo={} %GIDa_0b2e7fad_b81f_461a_8419_bb2a21777574
  wires:
  Switch1/1 -> Switch4/1
  [Out] -> Switch1/3
  Switch6/1 -> Switch1/1
  RelationalOperator1/1 -> Switch1/2
  K/1 -> RelationalOperator1/1, DetectSat1/2
  Constant1/1 -> RelationalOperator1/2
  LogicalOperator5/1 -> Switch4/2
  Switch4/1 -> sameDT2/2, UnitDelay1/1, Out/1
  Init/1 -> Switch4/3, sameDT2/3
  [In] -> sameDT2/1
  UnitDelay1/1 -> [Out]
  Switch7/1 -> Switch6/1
  Switch5/1 -> sameDT1/1, Switch6/3, RelationalOperator4/2, RelationalOperator6/1, Sum9/1, Sum8/1, UnitDelay2/1
  RelationalOperator7/1 -> Switch7/2
  [In] -> RelationalOperator7/1
  [Out1] -> RelationalOperator7/2
  Sum9/1 -> Switch7/3
  Sum8/1 -> Switch7/1
  LogicalOperator6/1 -> Switch6/2
  SIConvert/1 -> Sum8/2, sameDT1/2, Sum9/2
  Constant16/1 -> SIConvert/1
  RelationalOperator4/1 -> LogicalOperator6/2
  RelationalOperator6/1 -> LogicalOperator6/1
  [In] -> RelationalOperator6/2
  [In] -> RelationalOperator3/1
  [In] -> Sum6/2
  [In] -> Sum2/1
  In/1 -> [In]
  [Out1] -> RelationalOperator4/1
  Sum7/1 -> Switch5/3
  Sum6/1 -> Divide5/2
  [Out] -> Sum6/1
  Sum5/1 -> Switch5/1
  Sum2/1 -> Divide3/1
  RelationalOperator3/1 -> Switch5/2
  [Out1] -> RelationalOperator3/2
  [Out] -> Sum2/2
  Constant9/1 -> DetectSat1/1
  Constant10/1 -> DetectSat1/3
  DetectSat1/1 -> Divide3/2, Divide5/1
  LogicalOperator1/1 -> LogicalOperator5/1
  UnitDelay5/1 -> LogicalOperator5/2
  Rst/1 -> LogicalOperator1/1
  Constant11/1 -> UnitDelay5/1
  UnitDelay2/1 -> [Out1]
  Divide3/1 -> Sum5/2
  [Out] -> Sum5/1
  [Out] -> Sum7/1
  Divide5/1 -> Sum7/2

== system Valeo_Simulink_Library_EC/Signal_Operations/DKLowPassFilter_Float ==
  In : Inport
  Init : Inport  Port=2
  K : Inport  Port=3
  Rst : Inport  Port=4
  Constant1 : Constant  OutDataTypeStr=Inherit: Inherit via back propagation  SampleTime=-1
  Constant2 : Constant  Value=0  OutDataTypeStr=Inherit: Inherit via back propagation  SampleTime=-1
  Constant5 : Constant  OutDataTypeStr=boolean  SampleTime=-1
  DetectSat : Valeo_Simulink_Library_EC/Signal_Operations/DetectSat  FlagHitMax=off  FlagHitMin=off  FlagOut=on  FlagRevThr=off  EnableRevThreshold=No  LibType=Simulink_Library
  Divide2 : Product  Tag=struct('comment',struct('text','','placement',1),'logdata',struct('maxnumvals',inf,'plotchannels',[],'loggingmode',3,'channels',1),'output',struct('variable','','description','','name','$S_$B','width',1,'address','','max',NaN,'min',NaN,'class','default','type','CONTINUOUS','scaling','','lsb',1,'offset',0,'arb',0,'freeze',1,'unit','','autoscalingmode',1,'lowerheadroom',1,'upperheadroom',1,'headroomunit','bit','keepdatatype',1,'checkmin',0,'checkmax',0,'castoutput',0,'show',0),'inputs','**','exceptionhandling',1,'scalingvalid',0,'date',730486)  Inputs=**  OutDataTypeStr=Inherit: Inherit via back propagation  RndMeth=Nearest  SaturateOnIntegerOverflow=on  InputSameDT=on
  LogicalOperator2 : Logic  Operator=NOT  Inputs=1  OutDataTypeStr=boolean
  LogicalOperator3 : Logic  OutDataTypeStr=boolean
  Sum3 : Sum  Inputs=+-  OutDataTypeStr=Inherit: Inherit via back propagation  RndMeth=Nearest  SaturateOnIntegerOverflow=on  InputSameDT=on
  Sum4 : Sum  OutDataTypeStr=Inherit: Inherit via back propagation  RndMeth=Nearest  SaturateOnIntegerOverflow=on  InputSameDT=on
  Switch1 : Switch  Tag=struct('comment',struct('text','','placement',1),'logdata',struct('maxnumvals',inf,'plotchannels',[],'loggingmode',3,'channels',1),'output',struct('variable','','description','','name','$S_$B','width',1,'address','','max',NaN,'min',NaN,'class','default','type','CONTINUOUS','scaling','','lsb',1,'offset',0,'arb',0,'freeze',1,'unit','','autoscalingmode',1,'lowerheadroom',1,'upperheadroom',1,'headroomunit','bit','keepdatatype',1,'checkmin',0,'checkmax',0,'castoutput',0,'show',0),'threshold',struct('variable','','description','','name','$S_$B_threshold','width',1,'address','','max',NaN,'min',NaN,'class','default','type','CONTINUOUS','scaling','','lsb',1,'offset',0,'arb',0,'freeze',1,'unit','','keepdatatype',1,'value','0','scalar',0,'criteria',3),'scalingvalid',0,'date',733087.49614628474,'inheritscaling',0)  Criteria=u2 ~= 0  OutDataTypeStr=Inherit: Inherit via back propagation  SaturateOnIntegerOverflow=on  InputSameDT=on
      settings: AttributesFormatString=threshold=%<threshold>\nCriteria : %<Criteria>
  UnitDelay2 : UnitDelay  SampleTime=-1
      settings: AttributesFormatString=%<Name>\nTe = %<SampleTime>\nIni=%<X0>
  UnitDelay3 : UnitDelay  SampleTime=-1
      settings: AttributesFormatString=Te = %<SampleTime>\nIni=%<X0>
  Out : Outport
  wires:
  Switch1/1 -> Out/1, UnitDelay2/1
  Sum4/1 -> Switch1/1
  Divide2/1 -> Sum4/1
  Sum3/1 -> Divide2/1
  In/1 -> Sum3/1
  UnitDelay2/1 -> Sum4/2, Sum3/2
  Constant5/1 -> UnitDelay3/1
  Rst/1 -> LogicalOperator2/1
  UnitDelay3/1 -> LogicalOperator3/2
  LogicalOperator3/1 -> Switch1/2
  LogicalOperator2/1 -> LogicalOperator3/1
  Init/1 -> Switch1/3
  DetectSat/1 -> Divide2/2
  Constant2/1 -> DetectSat/3
  Constant1/1 -> DetectSat/1
  K/1 -> DetectSat/2

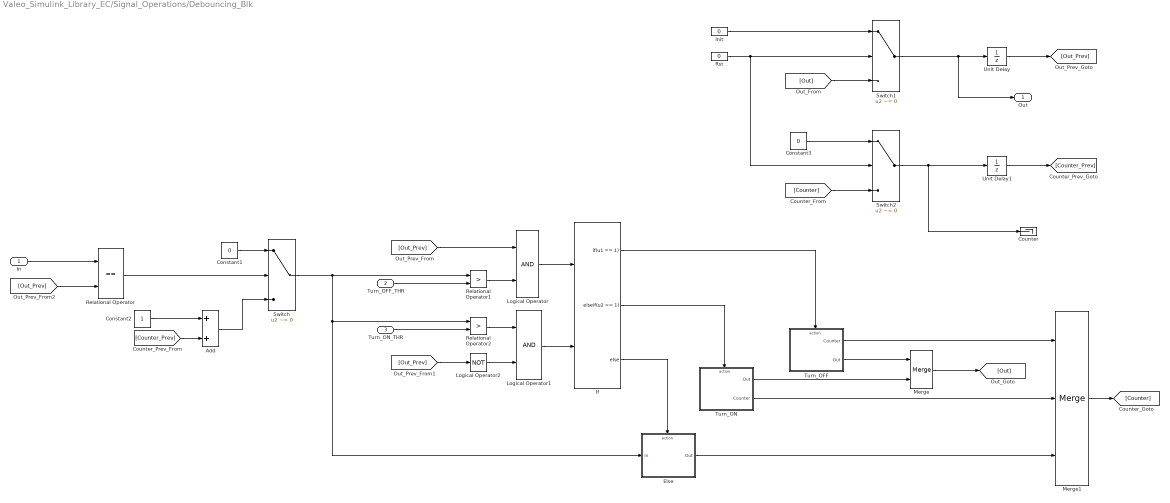
== system Valeo_Simulink_Library_EC/Signal_Operations/Debouncing_Blk ==
  In : Inport
  Turn_OFF_THR : Inport  Port=2
  Turn_ON_THR : Inport  Port=3
  Add : Sum  OutDataTypeStr=uint8  SaturateOnIntegerOverflow=on
  Constant1 : Constant  Value=0  OutDataTypeStr=uint8  SampleTime=-1
  Constant2 : Constant  OutDataTypeStr=uint8  SampleTime=-1
  Constant3 : Constant  Value=0  OutDataTypeStr=uint8  SampleTime=-1
  Counter : Terminator
  Else : Subsystem
  If : If  NumInputs=2  IfExpression=u1 == 1  ElseIfExpressions=u2 == 1
  Init : Constant  Value=0  OutDataTypeStr=boolean  SampleTime=-1
  Logical Operator : Logic  OutDataTypeStr=boolean
  Logical Operator1 : Logic  OutDataTypeStr=boolean
  Logical Operator2 : Logic  Operator=NOT  AllPortsSameDT=off  OutDataTypeStr=boolean
  Merge : Merge  InitialOutput=0
  Merge1 : Merge  Inputs=3
  Relational Operator : RelationalOperator  Operator===  OutDataTypeStr=boolean  RndMeth=Nearest
  Relational Operator1 : RelationalOperator  Operator=>  OutDataTypeStr=boolean  RndMeth=Nearest  InputSameDT=on
  Relational Operator2 : RelationalOperator  Operator=>  OutDataTypeStr=boolean  RndMeth=Nearest  InputSameDT=on
  Rst : Constant  Value=0  OutDataTypeStr=boolean  SampleTime=-1
  Switch : Switch  Criteria=u2 ~= 0
  Switch1 : Switch  Criteria=u2 ~= 0
  Switch2 : Switch  Criteria=u2 ~= 0
  Turn_OFF : Subsystem
  Turn_ON : Subsystem
  Unit Delay : UnitDelay  SampleTime=-1
  Unit Delay1 : UnitDelay  SampleTime=-1
  Out : Outport
  wires:
  Turn_OFF_THR/1 -> Relational Operator1/2
  Turn_ON_THR/1 -> Relational Operator2/2
  Relational Operator2/1 -> Logical Operator1/1
  Logical Operator2/1 -> Logical Operator1/2
  Logical Operator/1 -> If/1
  Turn_OFF/2(Out) -> Merge/1
  Turn_ON/1(Out) -> Merge/2
  Logical Operator1/1 -> If/2
  If/1 -> Turn_OFF/Action
  If/2 -> Turn_ON/Action
  Turn_OFF/1(Counter) -> Merge1/1
  Turn_ON/2(Counter) -> Merge1/2
  If/3 -> Else/Action
  Else/1(Out) -> Merge1/3
  In/1 -> Relational Operator/1
  Relational Operator1/1 -> Logical Operator/2
  Unit Delay/1 -> [Out_Prev]
  [Out_Prev] -> Logical Operator/1
  [Out_Prev] -> Logical Operator2/1
  [Out_Prev] -> Relational Operator/2
  Unit Delay1/1 -> [Counter_Prev]
  Switch/1 -> Relational Operator1/1, Else/1(In), Relational Operator2/1
  Relational Operator/1 -> Switch/2
  Constant2/1 -> Add/1
  [Counter_Prev] -> Add/2
  Add/1 -> Switch/3
  Constant1/1 -> Switch/1
  Switch1/1 -> Out/1, Unit Delay/1
  Merge/1 -> [Out]
  [Out] -> Switch1/3
  Init/1 -> Switch1/1
  Rst/1 -> Switch2/2, Switch1/2
  Constant3/1 -> Switch2/1
  Switch2/1 -> Counter/1, Unit Delay1/1
  Merge1/1 -> [Counter]
  [Counter] -> Switch2/3

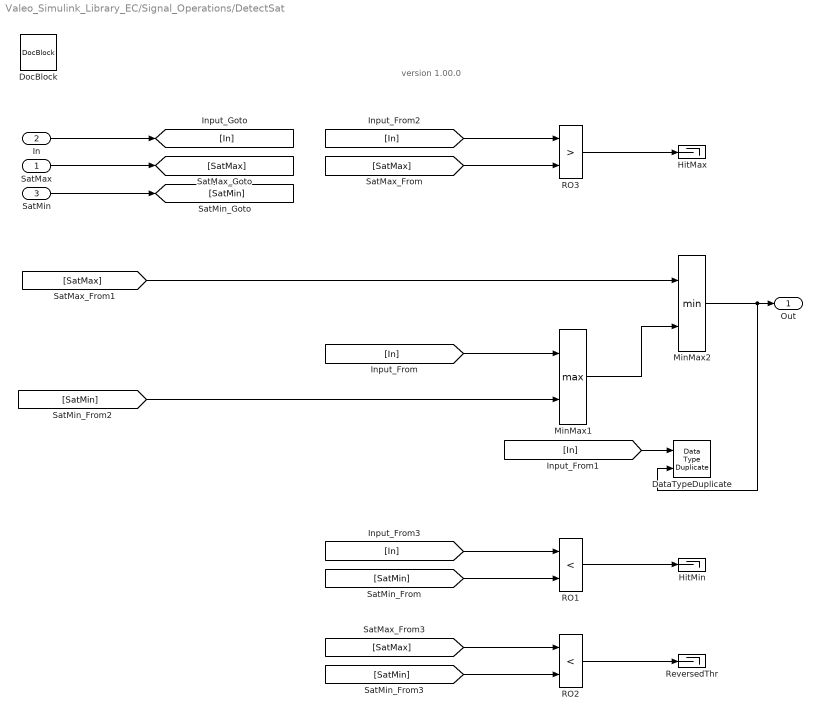
== system Valeo_Simulink_Library_EC/Signal_Operations/DetectSat ==
  note: version 1.00.0
  SatMax : Inport
  In : Inport  Port=2
  SatMin : Inport  Port=3
  DataTypeDuplicate : DataTypeDuplicate
  DocBlock : simulink/Model-Wide Utilities/DocBlock  DocumentType=Text
      content=|
      | BlockName: DetectSat
      |
      | Short Description: Saturation of Input Signal
      |
      | Requirements: {'SMBDP-REQ-0007(0)','SMBDP-REQ-0008(0)','SMBDP-REQ-0009(0)',
      | 'SMBDP-REQ-0010(0)','SMBDP-REQ-0011(0)','SMBDP-REQ-0012(0)','SMBDP-REQ-0013(0)',
      | 'SMBDP-REQ-0014(0)','SMBDP-REQ-0015(0)','SMBDP-REQ-0016(0)','SMBDP-REQ-0017(0)',
      | 'SMBDP-REQ-0018(0)'}
      |
      | Non-Functional Requirements: {'SMBDP-REQ-0001(0)','SMBDP-REQ-0002(0)',
      | 'SMBDP-REQ-0003(0)','SMBDP-REQ-0004(0)','SMBDP-REQ-0005(0)',
      | 'SMBDP-REQ-0022(0)','SMBDP-REQ-0006(0)'}
  HitMax : Terminator
  HitMin : Terminator
  MinMax1 : MinMax  RequirementInfo={} %GIDa_7ca5aa41_f951_487d_b293_f21b3bd29967  Function=max  Inputs=2  OutDataTypeStr=Inherit: Inherit via back propagation  RndMeth=Nearest  SaturateOnIntegerOverflow=on  InputSameDT=on
  MinMax2 : MinMax  RequirementInfo={} %GIDa_5d8bea90_416f_4184_af44_ef9f0c357b6b  Inputs=2  OutDataTypeStr=Inherit: Inherit via back propagation  RndMeth=Nearest  SaturateOnIntegerOverflow=on  InputSameDT=on
  RO1 : RelationalOperator  RequirementInfo={} %GIDa_6eb36581_c15a_41d6_b958_715c5ee5037f  Operator=<  OutDataTypeStr=boolean  ZeroCross=off  RndMeth=Nearest  InputSameDT=on
  RO2 : RelationalOperator  RequirementInfo={} %GIDa_551b4548_6028_477f_93e4_1ac37c1e0154  Operator=<  OutDataTypeStr=boolean  ZeroCross=off  RndMeth=Nearest  InputSameDT=on
  RO3 : RelationalOperator  RequirementInfo={} %GIDa_0a840635_fc62_4a1d_8ad0_d6ac649cc200  Operator=>  OutDataTypeStr=boolean  ZeroCross=off  RndMeth=Nearest  InputSameDT=on
  ReversedThr : Terminator
  Out : Outport
  wires:
  [SatMin] -> RO1/2
  [SatMax] -> RO3/2
  [SatMin] -> MinMax1/2
  [SatMax] -> MinMax2/1
  [In] -> RO1/1
  [In] -> RO3/1
  RO2/1 -> ReversedThr/1
  [SatMin] -> RO2/2
  [SatMax] -> RO2/1
  SatMin/1 -> [SatMin]
  SatMax/1 -> [SatMax]
  [In] -> DataTypeDuplicate/1
  [In] -> MinMax1/1
  In/1 -> [In]
  RO1/1 -> HitMin/1
  RO3/1 -> HitMax/1
  MinMax2/1 -> Out/1, DataTypeDuplicate/2
  MinMax1/1 -> MinMax2/2

== system Valeo_Simulink_Library_EC/Signal_Operations/FallingEdge ==
  In : Inport
  DocBlock1 : simulink/Model-Wide Utilities/DocBlock  DocumentType=Text
      content=|
      | Block Name: FallingEdge
      |
      | Description:
      | - Falling edge detection for a logic signal.
      | - When a falling edge on the input signal is detected, the output switches to 1 for only one computation period.
      | - Activation at initialization parameter (AAI) is used to activate the block at the Initialization.
      |
      |
      | Requirements Document:VIAS_T02_15_019_Valeo_Simulink_Library_SRS
      |                       Section:5.1.17
      |
      | Last Edit made by: sahmed1 on 27/5/2019
      |
      | Block Version: 1.1
  Logical : Logic  Tag=struct('inputs','2','comment',struct('text','','placement',1),'logdata',struct('maxnumvals',inf,'plotchannels',[],'loggingmode',3,'channels',1),'operator','AND','output',struct('variable','','description','','name','$S_$B','address','','class','default','type','Bool','unit',''),'scalingvalid',0,'date',733067.68453166669)  RequirementInfo={} %GIDa_afbf01c3_7d5e_49d9_9fca_fc074698d4a3  OutDataTypeStr=boolean
  Logical1 : Logic  Tag=struct('inputs','1','comment',struct('text','','placement',1),'logdata',struct('maxnumvals',inf,'plotchannels',[],'loggingmode',3,'channels',1),'operator','NOT','output',struct('variable','','description','','name','$S_$B','address','','class','default','type','Bool','unit',''),'scalingvalid',0,'date',733067.68453201384)  Operator=NOT  Inputs=1  OutDataTypeStr=boolean
  UnitDelay : UnitDelay  RequirementInfo={} %GIDa_38b5e67e_1674_42fb_82fd_b1aea6e8acb5  InitialCondition=Init  SampleTime=-1
      settings: AttributesFormatString=%<Name>\nTe = %<SampleTime>\nIni=%<X0>
  Out : Outport  OutDataTypeStr=boolean
  wires:
  UnitDelay/1 -> Logical/2
  Logical1/1 -> Logical/1
  In/1 -> UnitDelay/1, Logical1/1
  Logical/1 -> Out/1

== system Valeo_Simulink_Library_EC/Signal_Operations/KalmanFilter_single ==
  u : Inport  OutDataTypeStr=single
  y : Inport  Port=2  OutDataTypeStr=single
  Correct : Subsystem  RequirementInfo={} %GIDa_190862df_144c_4cbb_ab2c_0fd8a8001bf4
  Predict : Subsystem  RequirementInfo={} %GIDa_52eec7c0_a659_4e8b_b981_b004d00cd39c
  Terminator : Terminator
  Unit Delay1 : UnitDelay  InitialCondition=x0  SampleTime=-1
  Unit Delay3 : UnitDelay  InitialCondition=p0  SampleTime=-1
  Xhat : Outport
  wires:
  Unit Delay3/1 -> Predict/2(Pk-1)
  Correct/1(Pk) -> Unit Delay3/1, Terminator/1
  Predict/2(Xk_priori) -> Correct/4(Xk_priori)
  Predict/1(Pk_priori) -> Correct/3(Pk_priori)
  Unit Delay1/1 -> Predict/3(Xk-1)
  Correct/2(Xk) -> Unit Delay1/1, Xhat/1
  y/1 -> Correct/2(Yk)
  u/1 -> Predict/1(u), Correct/1(u)

== system Valeo_Simulink_Library_EC/Signal_Operations/Mem ==
  In : Inport
  Hld : Inport  Port=2  OutDataTypeStr=boolean
  DataTypeDuplicate : DataTypeDuplicate
  Switch : Switch  Tag=struct('comment',struct('text','','placement',1),'logdata',struct('maxnumvals',inf,'plotchannels',[],'loggingmode',3,'channels',1),'output',struct('variable','','description','','name','$S_$B','width',1,'address','','max',NaN,'min',NaN,'class','default','type','CONTINUOUS','scaling','','lsb',1,'offset',0,'arb',0,'freeze',1,'unit','','autoscalingmode',1,'lowerheadroom',1,'upperheadroom',1,'headroomunit','bit','keepdatatype',1,'checkmin',0,'checkmax',0,'castoutput',0,'show',0),'threshold',struct('variable','','description','','name','$S_$B_threshold','width',1,'address','','max',NaN,'min',NaN,'class','default','type','CONTINUOUS','scaling','','lsb',1,'offset',0,'arb',0,'freeze',1,'unit','','keepdatatype',1,'value','0','scalar',0,'criteria',3),'scalingvalid',0,'date',733087.49614628474,'inheritscaling',0)  Criteria=u2 ~= 0  OutDataTypeStr=Inherit: Inherit via back propagation  SaturateOnIntegerOverflow=on  InputSameDT=on
      settings: AttributesFormatString=threshold=%<threshold>\nCriteria : %<Criteria>
  UnitDelay : UnitDelay  InitialCondition=InitVal  SampleTime=-1
      settings: AttributesFormatString=%<Name>\nTe = %<SampleTime>\nIni=%<X0>
  Out : Outport
  wires:
  In/1 -> DataTypeDuplicate/2, Switch/3
  Switch/1 -> DataTypeDuplicate/1, Out/1, UnitDelay/1
  Hld/1 -> Switch/2
  UnitDelay/1 -> Switch/1

== system Valeo_Simulink_Library_EC/Signal_Operations/NegHys ==
  High : Inport
  In : Inport  Port=2
  Low : Inport  Port=3
  DataTypeDuplicate : DataTypeDuplicate  NumInputPorts=3
  Hysteresis : Subsystem  Description=Hysteresis  RTWFileName=sal_math
      settings: RTWSystemCode=Inline  RTWFcnNameOpts=Use subsystem name  RTWFileNameOpts=User specified
  UnitDelay : UnitDelay  SampleTime=-1
  Out : Outport
  wires:
  UnitDelay/1 -> Hysteresis/4(RemainderIN)
  Hysteresis/1(Out) -> Out/1, UnitDelay/1
  Low/1 -> DataTypeDuplicate/1, Hysteresis/1(Low)
  In/1 -> DataTypeDuplicate/2, Hysteresis/2(In)
  High/1 -> DataTypeDuplicate/3, Hysteresis/3(High)

== system Valeo_Simulink_Library_EC/Signal_Operations/PosHys ==
  High : Inport
  In : Inport  Port=2
  Low : Inport  Port=3
  DataTypeDuplicate : DataTypeDuplicate  NumInputPorts=3
  Hysteresis : Subsystem  Description=Hysteresis  RTWFileName=sal_math
      settings: RTWSystemCode=Inline  RTWFcnNameOpts=Use subsystem name  RTWFileNameOpts=User specified
  UnitDelay : UnitDelay  SampleTime=-1
  Out : Outport
  wires:
  Hysteresis/1(Out) -> Out/1, UnitDelay/1
  UnitDelay/1 -> Hysteresis/4(RemainderIN)
  Low/1 -> DataTypeDuplicate/3, Hysteresis/1(Low)
  In/1 -> DataTypeDuplicate/2, Hysteresis/2(In)
  High/1 -> DataTypeDuplicate/1, Hysteresis/3(High)

== system Valeo_Simulink_Library_EC/Signal_Operations/RisingEdge ==
  In : Inport
  DocBlock : simulink/Model-Wide Utilities/DocBlock  DocumentType=Text
      content=|
      | Block Name: RisingEdge
      |
      | Description:
      | - Rising edge detection for a logic signal.
      | - When a rising edge on the input signal is detected, the output switches to 1 for only one computation period.
      | - Activation at initialization parameter (AAI) is used to activate the block at the Initialization.
      |
      |
      | Requirements Document:VIAS_T02_15_019_Valeo_Simulink_Library_SRS
      |                       Section:5.1.3
      |
      | Last Edit made by: sahmed1 on 16/4/2019
      |
      | Block Version: 1.1
  LogicalOperator : Logic  Tag=struct('inputs','2','comment',struct('text','','placement',1),'logdata',struct('maxnumvals',inf,'plotchannels',[],'loggingmode',3,'channels',1),'operator','AND','output',struct('variable','','description','','name','$S_$B','address','','class','default','type','Bool','unit',''),'scalingvalid',0,'date',733067.68458487268)  RequirementInfo={} %GIDa_46b4697c_c428_4231_8e35_ed6f95728904  OutDataTypeStr=boolean
  LogicalOperator1 : Logic  Tag=struct('inputs','1','comment',struct('text','','placement',1),'logdata',struct('maxnumvals',inf,'plotchannels',[],'loggingmode',3,'channels',1),'operator','NOT','output',struct('variable','','description','','name','$S_$B','address','','class','default','type','Bool','unit',''),'scalingvalid',0,'date',733067.68458533566)  Operator=NOT  Inputs=1  OutDataTypeStr=boolean
  UnitDelay : UnitDelay  RequirementInfo={} %GIDa_e97586d9_635f_41d8_ab1f_7563d0e0a8e3  InitialCondition=Init  SampleTime=-1
  Out : Outport  OutDataTypeStr=boolean
  wires:
  UnitDelay/1 -> LogicalOperator/2
  LogicalOperator1/1 -> UnitDelay/1
  LogicalOperator/1 -> Out/1
  In/1 -> LogicalOperator/1, LogicalOperator1/1

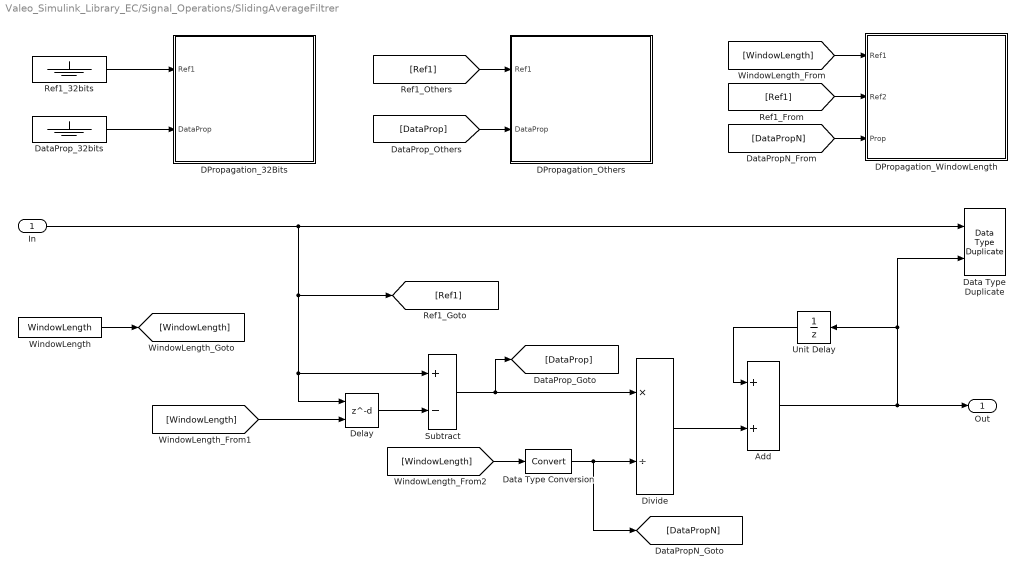
== system Valeo_Simulink_Library_EC/Signal_Operations/SlidingAverageFiltrer ==
  In : Inport
  Add : Sum  OutDataTypeStr=Inherit: Inherit via back propagation  RndMeth=Nearest  SaturateOnIntegerOverflow=on
  DPropagation_32Bits : Subsystem
  DPropagation_Others : Subsystem
  DPropagation_WindowLength : Subsystem
  Data Type Duplicate : DataTypeDuplicate
  Data Type Conversion : DataTypeConversion
  DataProp_32bits : Ground
  Delay : Delay  DelayLengthSource=Input port  DelayLength=Length  DelayLengthUpperLimit=WindowLength  InitialCondition=0
      settings: InputPortMap=u0,p1
  Divide : Product  Inputs=*/  RndMeth=Nearest  OutDataTypeStr=Inherit: Same as first input
  Ref1_32bits : Ground
  Subtract : Sum  Inputs=+-  OutDataTypeStr=Inherit: Inherit via back propagation  RndMeth=Nearest  SaturateOnIntegerOverflow=on
  Unit Delay : UnitDelay  SampleTime=-1
  WindowLength : Constant  Value=WindowLength  OutDataTypeStr=Inherit: Inherit via back propagation  SampleTime=-1
  Out : Outport
  wires:
  Add/1 -> Out/1, Unit Delay/1, Data Type Duplicate/2
  Delay/1 -> Subtract/2
  Divide/1 -> Add/2
  Unit Delay/1 -> Add/1
  In/1 -> [Ref1], Subtract/1, Delay/1, Data Type Duplicate/1
  Subtract/1 -> [DataProp], Divide/1
  [Ref1] -> DPropagation_Others/1(Ref1)
  [DataProp] -> DPropagation_Others/2(DataProp)
  Ref1_32bits/1 -> DPropagation_32Bits/1(Ref1)
  DataProp_32bits/1 -> DPropagation_32Bits/2(DataProp)
  WindowLength/1 -> [WindowLength]
  [WindowLength] -> Delay/2
  [WindowLength] -> Data Type Conversion/1
  [WindowLength] -> DPropagation_WindowLength/1(Ref1)
  [Ref1] -> DPropagation_WindowLength/2(Ref2)
  Data Type Conversion/1 -> [DataPropN], Divide/2
  [DataPropN] -> DPropagation_WindowLength/3(Prop)
